simulink model "bus_test"  (Simulink 8.4)
settings: Solver=ode45  StartTime=0.0  StopTime=10.0  RelTol=1e-3
undefined symbols (not defined in the file): signal1, signal3
settings Model: Creator=arnaud  LastModifiedBy=arnaud
settings DataIOCC: SaveFormat=StructureWithTime

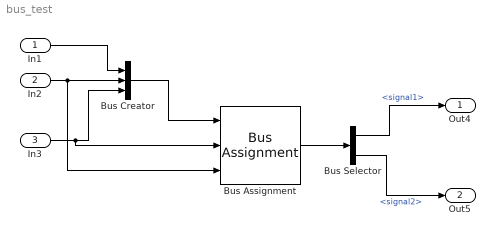
== system bus_test ==
  In1 : Inport  PortDimensions=1
  In2 : Inport  Port=2  PortDimensions=1
  In3 : Inport  Port=3  OutDataTypeStr=double  PortDimensions=1
  Bus Assignment : BusAssignment  AssignedSignals=signal1,signal3
  Bus Creator : BusCreator  Inputs=3
  Bus Selector : BusSelector  OutputSignals=signal1,signal2
  Out4 : Outport
  Out5 : Outport  Port=2
  wires:
  In2/1 -> Bus Creator/2, Bus Assignment/3
  In3/1 -> Bus Assignment/2, Bus Creator/3
  In1/1 -> Bus Creator/1
  Bus Creator/1 -> Bus Assignment/1
  Bus Selector/1 -> Out4/1  "<signal1>"
  Bus Selector/2 -> Out5/1  "<signal2>"
  Bus Assignment/1 -> Bus Selector/1
